simulink model "time_gongji_daoyuan"  (R2019b)
settings: Solver=ode3  StartTime=0.0  StopTime=6000  FixedStep=0.01  MaxStep=0.01  RelTol=1e-3
values from neighbouring files (symbols this model uses):
  bias_gyro_z_gongji = -0.7e-3    (= -0.0007)    [sych_ite_KVHpost_daoyuan_huace.m]
  g = 9.8    [sych_ite_KVHpost_daoyuan_huace.m]
settings Model: Creator=luyishi_E480  LastModifiedBy=xie_z
settings DataIOCC: SaveOutput=off  SignalLogging=off  DSMLogging=off  InspectSignalLogs=on  SaveTime=off  ReturnWorkspaceOutputs=off
settings DebuggingCC: InheritedTsInSrcMsg=none

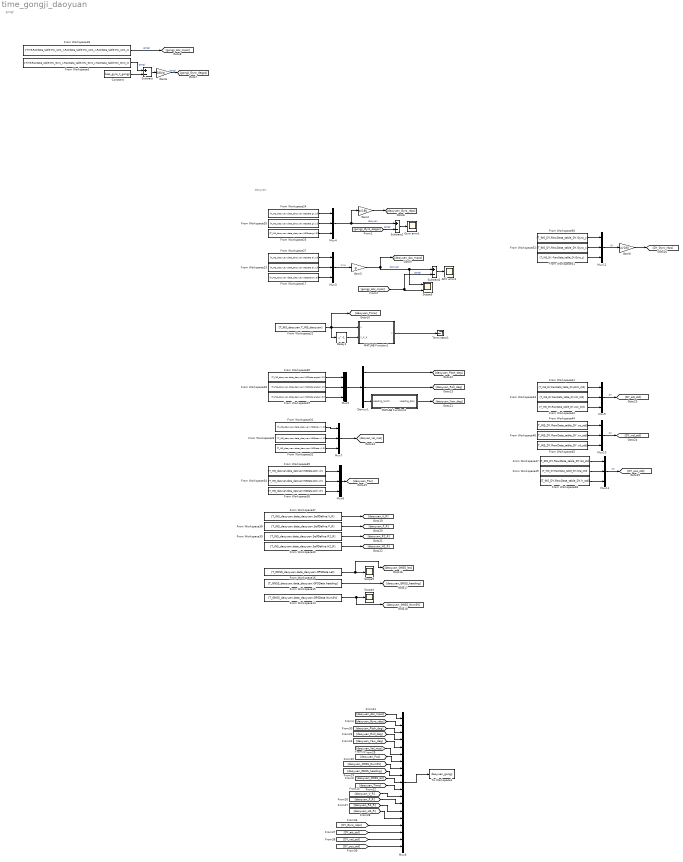
== system time_gongji_daoyuan ==
  note: daoyuan
  note: gongji
  ACC error1 : Scope
  Constant : Constant  Value=bias_gyro_z_gongji
  Delay1 : Delay  DelayLength=1  InitialCondition=0
  Demux1 : Demux  Outputs=3
  From Workspace14 : FromWorkspace  VariableName=[T_GNSS_daoyuan,data_daoyuan.GPSData.NumSV]  Interpolate=off  OutputAfterFinalValue=Holding final value
  From Workspace15 : FromWorkspace  VariableName=[T_GNSS_daoyuan,data_daoyuan.GPSData.heading]  Interpolate=off  OutputAfterFinalValue=Holding final value
  From Workspace16 : FromWorkspace  VariableName=[T_GNSS_daoyuan,data_daoyuan.GPSData.Lat]  Interpolate=off  OutputAfterFinalValue=Holding final value
  From Workspace17 : FromWorkspace  VariableName=[T_INS_daoyuan,-data_daoyuan.INSData.a(:,3)]  Interpolate=off  OutputAfterFinalValue=Holding final value
  From Workspace18 : FromWorkspace  VariableName=[Time,RawData_table.IMU_ACC_x,RawData_table.IMU_ACC_y,RawData_table.IMU_ACC_z]  Interpolate=off  OutputAfterFinalValue=Holding final value
  From Workspace2 : FromWorkspace  VariableName=[Time,RawData_table.IMU_Gyro_x,RawData_table.IMU_Gyro_y,RawData_table.IMU_Gyro_z]  Interpolate=off  OutputAfterFinalValue=Holding final value
  From Workspace22 : FromWorkspace  VariableName=[T_INS_daoyuan,T_INS_daoyuan]  Interpolate=off  OutputAfterFinalValue=Holding final value
  From Workspace23 : FromWorkspace  VariableName=[T_INS_daoyuan,data_daoyuan.INSData.a(:,1)]  Interpolate=off  OutputAfterFinalValue=Holding final value
  From Workspace24 : FromWorkspace  VariableName=[T_INS_daoyuan,data_daoyuan.INSData.g(:,2)]  Interpolate=off  OutputAfterFinalValue=Holding final value
  From Workspace25 : FromWorkspace  VariableName=[T_INS_daoyuan,-data_daoyuan.INSData.g(:,3)]  Interpolate=off  OutputAfterFinalValue=Holding final value
  From Workspace26 : FromWorkspace  VariableName=[T_INS_daoyuan,data_daoyuan.INSData.g(:,1)]  Interpolate=off  OutputAfterFinalValue=Holding final value
  From Workspace27 : FromWorkspace  VariableName=[T_INS_daoyuan,data_daoyuan.INSData.a(:,2)]  Interpolate=off  OutputAfterFinalValue=Holding final value
  From Workspace28 : FromWorkspace  VariableName=[T_INS_daoyuan,data_daoyuan.INSData.angle(:,1)]  Interpolate=off  OutputAfterFinalValue=Holding final value
  From Workspace29 : FromWorkspace  VariableName=[T_INS_daoyuan,data_daoyuan.INSData.angle(:,3)]  Interpolate=off  OutputAfterFinalValue=Holding final value
  From Workspace30 : FromWorkspace  VariableName=[T_INS_daoyuan,data_daoyuan.INSData.angle(:,2)]  Interpolate=off  OutputAfterFinalValue=Holding final value
  From Workspace31 : FromWorkspace  VariableName=[T_INS_daoyuan,data_daoyuan.INSData.v(:,2)]  Interpolate=off  OutputAfterFinalValue=Holding final value
  From Workspace32 : FromWorkspace  VariableName=[T_INS_daoyuan,-data_daoyuan.INSData.v(:,3)]  Interpolate=off  OutputAfterFinalValue=Holding final value
  From Workspace33 : FromWorkspace  VariableName=[T_INS_daoyuan,data_daoyuan.INSData.v(:,1)]  Interpolate=off  OutputAfterFinalValue=Holding final value
  From Workspace34 : FromWorkspace  VariableName=[T_INS_daoyuan,data_daoyuan.INSData.pos(:,2)]  Interpolate=off  OutputAfterFinalValue=Holding final value
  From Workspace35 : FromWorkspace  VariableName=[T_INS_daoyuan,data_daoyuan.INSData.pos(:,1)]  Interpolate=off  OutputAfterFinalValue=Holding final value
  From Workspace36 : FromWorkspace  VariableName=[T_INS_daoyuan,data_daoyuan.INSData.pos(:,3)]  Interpolate=off  OutputAfterFinalValue=Holding final value
  From Workspace37 : FromWorkspace  VariableName=[T_INS_daoyuan,data_daoyuan.SelfDefine.V_R]  Interpolate=off  OutputAfterFinalValue=Holding final value
  From Workspace38 : FromWorkspace  VariableName=[T_INS_daoyuan,data_daoyuan.SelfDefine.P_R]  Interpolate=off  OutputAfterFinalValue=Holding final value
  From Workspace39 : FromWorkspace  VariableName=[T_INS_daoyuan,data_daoyuan.SelfDefine.R2_R]  Interpolate=off  OutputAfterFinalValue=Holding final value
  From Workspace40 : FromWorkspace  VariableName=[T_INS_daoyuan,data_daoyuan.SelfDefine.H2_R]  Interpolate=off  OutputAfterFinalValue=Holding final value
  From Workspace41 : FromWorkspace  VariableName=[T_INS_DY,RawData_table_DY.pitch_std]  Interpolate=off  OutputAfterFinalValue=Holding final value
  From Workspace42 : FromWorkspace  VariableName=[T_INS_DY,RawData_table_DY.yaw_std]  Interpolate=off  OutputAfterFinalValue=Holding final value
  From Workspace43 : FromWorkspace  VariableName=[T_INS_DY,RawData_table_DY.roll_std]  Interpolate=off  OutputAfterFinalValue=Holding final value
  From Workspace44 : FromWorkspace  VariableName=[T_INS_DY,RawData_table_DY.ve_std]  Interpolate=off  OutputAfterFinalValue=Holding final value
  From Workspace45 : FromWorkspace  VariableName=[T_INS_DY,RawData_table_DY.vd_std]  Interpolate=off  OutputAfterFinalValue=Holding final value
  From Workspace46 : FromWorkspace  VariableName=[T_INS_DY,RawData_table_DY.vn_std]  Interpolate=off  OutputAfterFinalValue=Holding final value
  From Workspace47 : FromWorkspace  VariableName=[T_INS_DY,RawData_table_DY.lat_std]  Interpolate=off  OutputAfterFinalValue=Holding final value
  From Workspace48 : FromWorkspace  VariableName=[T_INS_DY,RawData_table_DY.h_std]  Interpolate=off  OutputAfterFinalValue=Holding final value
  From Workspace49 : FromWorkspace  VariableName=[T_INS_DY,RawData_table_DY.long_std]  Interpolate=off  OutputAfterFinalValue=Holding final value
  From Workspace50 : FromWorkspace  VariableName=[T_INS_DY,RawData_table_DY.Gyro_y]  Interpolate=off  OutputAfterFinalValue=Holding final value
  From Workspace51 : FromWorkspace  VariableName=[T_INS_DY,-RawData_table_DY.Gyro_z]  Interpolate=off  OutputAfterFinalValue=Holding final value
  From Workspace52 : FromWorkspace  VariableName=[T_INS_DY,RawData_table_DY.Gyro_x]  Interpolate=off  OutputAfterFinalValue=Holding final value
  Gain2 : Gain  Gain=pi/180
  Gain3 : Gain  Gain=g
  Gain6 : Gain  Gain=180/pi
  Gain8 : Gain  Gain=pi/180
  Gyro error1 : Scope
  MATLAB Function1 : MATLAB Function  TreatAsAtomicUnit=on
  MATLAB Function3 : MATLAB Function  TreatAsAtomicUnit=on
  Mux{3..5,7..12} (9 alike) : Mux  Inputs=3
  Mux6 : Mux  Inputs=19
  Scope3 : Scope  NumInputPorts=2
  Scope4 : Scope
  Scope5 : Scope
  Subtract : Sum  Inputs=+-
  Subtract1 : Sum  Inputs=+-
  Subtract2 : Sum  Inputs=+-
  Terminator1 : Terminator
  To Workspace1 : ToWorkspace  VariableName=daoyuan_gongji  SaveFormat=Structure With Time  SampleTime=-1
  wires:
  Subtract/1 -> Gain6/1
  Constant/1 -> Subtract/2
  From Workspace2/1 -> Subtract/1  "gongji"
  From Workspace18/1 -> [gongji_Acc_mpss]  "gongji"
  Gain6/1 -> [gongji_Gyro_degps]  "gongji"
  [gongji_Acc_mpss] -> Subtract2/2, Scope3/2  "gongji"
  From Workspace25/1 -> Mux4/3
  From Workspace23/1 -> Mux3/2
  Mux3/1 -> Gain3/1  "KVH"
  [gongji_Gyro_degps] -> Subtract1/2  "gongji"
  Gain3/1 -> [daoyuan_Acc_mpss], Scope3/1, Subtract2/1  "daoyuan"
  Mux4/1 -> Gain2/1, Subtract1/1  "daoyuan"
  From Workspace17/1 -> Mux3/3
  Gain2/1 -> [daoyuan_Gyro_rdps]
  From Workspace24/1 -> Mux4/1
  From Workspace27/1 -> Mux3/1
  Subtract2/1 -> ACC error1/1
  Delay1/1 -> MATLAB Function1/2(x_k_1)
  MATLAB Function1/1(y) -> Terminator1/1
  From Workspace26/1 -> Mux4/2
  Subtract1/1 -> Gyro error1/1
  From Workspace22/1 -> [daoyuan_Time], Delay1/1, MATLAB Function1/1(x)
  MATLAB Function3/1(Heading_ENU) -> [daoyuan_Yaw_deg]
  Demux1/3 -> MATLAB Function3/1(Heading_North)
  Mux5/1 -> Demux1/1
  Demux1/1 -> [daoyuan_Pitch_deg]
  From Workspace30/1 -> Mux5/1
  Demux1/2 -> [daoyuan_Roll_deg]
  From Workspace29/1 -> Mux5/3
  From Workspace28/1 -> Mux5/2
  [DY_Gyro_rdps] -> Mux6/16
  [daoyuan_H2_R] -> Mux6/15
  [daoyuan_P_R] -> Mux6/13
  [daoyuan_GNSS_lat] -> Mux6/10
  [daoyuan_V_R] -> Mux6/12
  [daoyuan_Yaw_deg] -> Mux6/5
  [daoyuan_Vel_mps] -> Mux6/6
  [daoyuan_Pitch_deg] -> Mux6/3
  [daoyuan_Roll_deg] -> Mux6/4
  [daoyuan_R2_R] -> Mux6/14
  [daoyuan_GNSS_heading] -> Mux6/9
  [DY_vel_std] -> Mux6/18
  [daoyuan_GNSS_NumSV] -> Mux6/8
  [daoyuan_Time] -> Mux6/11
  [daoyuan_Pos] -> Mux6/7
  [daoyuan_Acc_mpss] -> Mux6/1
  [daoyuan_Gyro_rdps] -> Mux6/2
  [DY_att_std] -> Mux6/17
  [DY_pos_std] -> Mux6/19
  Mux6/1 -> To Workspace1/1
  From Workspace33/1 -> Mux7/2
  From Workspace31/1 -> Mux7/1
  Mux7/1 -> [daoyuan_Vel_mps]
  From Workspace32/1 -> Mux7/3
  From Workspace34/1 -> Mux8/2
  From Workspace35/1 -> Mux8/1
  Mux8/1 -> [daoyuan_Pos]
  From Workspace36/1 -> Mux8/3
  From Workspace14/1 -> [daoyuan_GNSS_NumSV], Scope4/1
  From Workspace15/1 -> [daoyuan_GNSS_heading]
  From Workspace16/1 -> Scope5/1, [daoyuan_GNSS_lat]
  From Workspace38/1 -> [daoyuan_P_R]
  From Workspace40/1 -> [daoyuan_H2_R]
  From Workspace39/1 -> [daoyuan_R2_R]
  From Workspace37/1 -> [daoyuan_V_R]
  From Workspace44/1 -> Mux10/1
  From Workspace48/1 -> Mux11/3
  From Workspace45/1 -> Mux10/3
  Mux11/1 -> [DY_pos_std]  "DY"
  Mux10/1 -> [DY_vel_std]  "DY"
  From Workspace49/1 -> Mux11/2
  From Workspace47/1 -> Mux11/1
  From Workspace42/1 -> Mux9/3
  From Workspace46/1 -> Mux10/2
  From Workspace41/1 -> Mux9/1
  Mux9/1 -> [DY_att_std]  "DY"
  From Workspace43/1 -> Mux9/2
  From Workspace51/1 -> Mux12/3
  From Workspace52/1 -> Mux12/2
  Mux12/1 -> Gain8/1  "DY"
  Gain8/1 -> [DY_Gyro_rdps]
  From Workspace50/1 -> Mux12/1

== matlab function time_gongji_daoyuan/MATLAB Function1 ==
  data: y output; x input; x_k_1 input
function y  = fcn(x,x_k_1)
    if x ~= x_k_1
        y = uint8(1);
    else
        y = uint8(0);
    end
end

== matlab function time_gongji_daoyuan/MATLAB Function3 ==
  data: Heading_North input; Heading_ENU output size=1
function Heading_ENU = fcn(Heading_North)
% Heading_ENU:以北为零顺时针为正0-360°
% Heading_North:以北为零逆时针为正-180-180°

% Heading_North = Heading_North + 0.5 + 3.8;
if Heading_North <= 180
    Heading_ENU = 0 - Heading_North;
else
    Heading_ENU = 360 - Heading_North;
end
